simulink model "level0"  (R2018a)
settings: Solver=VariableStepAuto  StartTime=0.0  StopTime=10  RelTol=1e-3
settings Model: Creator=gonzalo  LastModifiedBy=gonzalo

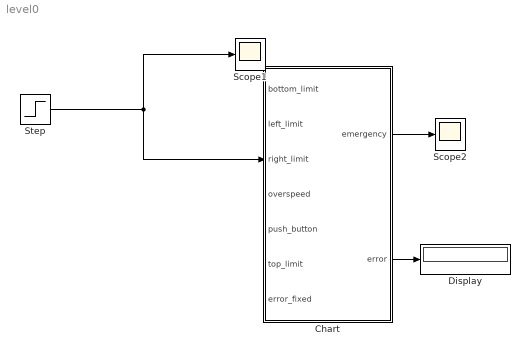
== system level0 ==
  Chart : Stateflow chart  TreatAsAtomicUnit=on
  Display : Display
  Scope1 : Scope
  Scope2 : Scope
  Step : Step  Time=2  SampleTime=0
  wires:
  Chart/1(emergency) -> Scope2/1
  Step/1 -> Chart/3(right_limit), Scope1/1
  Chart/2(error) -> Display/1

== stateflow chart level0/Chart ==
  state Level_0
    state Emergency_limit_switch_horizontal
      entry:
      emergency = 1;
      if (bottom_limit == 1)
      error = 1;
      else
      error = 2;
      end
    state Normal
      entry:
      emergency = 0;
      error = 0;
    state Emergency_limit_switch_vertical
      entry:
      emergency = 1;
      if (bottom_limit == 1)
      error = 3;
      else
      error = 4;
      end
    state Emergency_overspeed
      entry:
      emergency = 1;
      error = 5;
    state Emergency_button
      entry:
      emergency = 1;
      error = 6;
    Normal -> Emergency_limit_switch_horizontal [order 1] : [(right_limit == 1)||(left_limit == 1)]
    Normal -> Emergency_limit_switch_vertical [order 2] : [(top_limit == 1) || (bottom_limit == 1)]
    (default) -> Normal
    Normal -> Emergency_overspeed [order 4] : [overspeed == 1]
    Normal -> Emergency_button [order 3] : [push_button == 1]
  state Emergency
    state emergency_handler
      during:
      %emergency_routine()
    state end_emergency
      entry:
      %check_security()
      emergency = 0
    (default) -> emergency_handler
    emergency_handler -> end_emergency : [error_fixed == 1]
  (default) -> Level_0
  Level_0 -> Emergency : [emergency == 1]
  Emergency -> Level_0 : [emergency == 0]
  data: bottom_limit input; left_limit input; right_limit input; overspeed input; push_button input; top_limit input; emergency output; error output; error_fixed input
